simulink model "Isolette"  (R2020a)
settings: Solver=VariableStepAuto  StartTime=0.0  StopTime=200  RelTol=1e-3
settings Model: Creator=BEAR  LastModifiedBy=bzhan
settings DataIOCC: ReturnWorkspaceOutputs=off
settings DebuggingCC: ArithmeticOperatorsInVariantConditions=warning
settings SFSimCC: SimUseLocalCustomCode=off  CustomCodeUndefinedFunction=UseInterfaceOnly
settings RTWCC: RTWUseLocalCustomCode=off

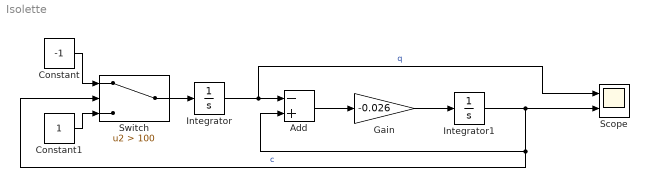
== system Isolette ==
  Add : Sum  Inputs=-+
  Constant : Constant  Value=-1
  Constant1 : Constant
  Gain : Gain  Gain=-0.026
  Integrator : Integrator  InitialCondition=75
  Integrator1 : Integrator  InitialCondition=75
  Scope : Scope  NumInputPorts=2
  Switch : Switch  Criteria=u2 > Threshold  Threshold=100
  wires:
  Constant/1 -> Switch/1
  Switch/1 -> Integrator/1
  Integrator/1 -> Scope/1, Add/1  "q"
  Add/1 -> Gain/1
  Gain/1 -> Integrator1/1
  Constant1/1 -> Switch/3
  Integrator1/1 -> Scope/2, Add/2, Switch/2  "c"
